simulink model "Fig7_Control_RLcurrent_PI"  (R2022a)
settings: Solver=FixedStepAuto  StartTime=0.0  StopTime=0.4  FixedStep=1e-4  RelTol=1e-3
InitFcn:
  | KpKiDesign
StartFcn:
  | KpKiDesign
values from neighbouring files (symbols this model uses):
  Ki = R/tau    (= 5)    [Fig17_drawBodeCPminusP.m]    (also in Fig22_drawBodePIctrl.m = [0.1;  0;      0;      0.1; 0.1]; KpKiDesign.m)
  Kp = L/tau    (= 0.2)    [Fig17_drawBodeCPminusP.m]    (also in Fig22_drawBodePIctrl.m = [0;    0.01;   0.1;    0.1; 0.01]; KpKiDesign.m)
  L = 4e-3    (= 0.004)    [Fig17_drawBodeCPminusP.m]    (also in KpKiDesign.m; RLCurcuitParam.m)
  R = 0.1    [Fig17_drawBodeCPminusP.m]    (also in KpKiDesign.m; RLCurcuitParam.m)
settings Model: Creator=r720r  LastModifiedBy=r720r

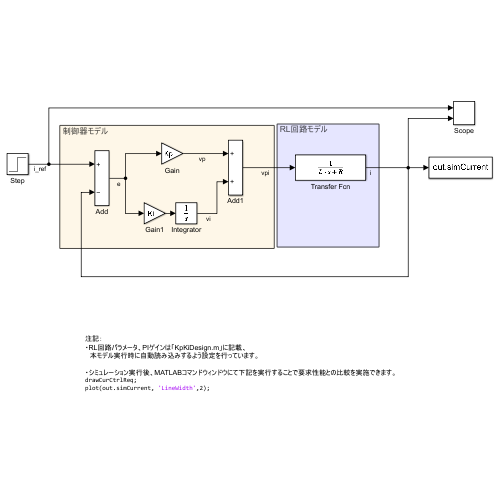
[thumbnail: Simulink's stored preview of the top-level diagram]
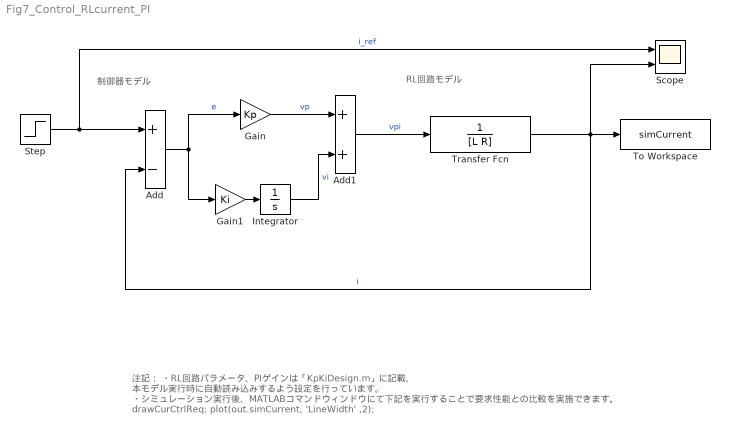
== system Fig7_Control_RLcurrent_PI ==
  note: RL回路モデル
  note: 制御器モデル
  note: 注記：
      | ・RL回路パラメータ、PIゲインは「KpKiDesign.m」に記載、
      | 本モデル実行時に自動読み込みするよう設定を行っています。
      |
      | ・シミュレーション実行後、MATLABコマンドウィンドウにて下記を実行することで要求性能との比較を実施できます。
      | drawCurCtrlReq;
      | plot(out.simCurrent, 'LineWidth' ,2);
  Add : Sum  Inputs=+-
  Add1 : Sum
  Gain : Gain  Gain=Kp
  Gain1 : Gain  Gain=Ki
  Integrator : Integrator
  Scope : Scope  NumInputPorts=2
  Step : Step  Time=0  SampleTime=0
  To Workspace : ToWorkspace  VariableName=simCurrent  SaveFormat=Timeseries  SampleTime=-1
  Transfer Fcn : TransferFcn  Denominator=[L R]
  wires:
  Step/1 -> Scope/1, Add/1  "i_ref"
  Add/1 -> Gain/1, Gain1/1  "e"
  Transfer Fcn/1 -> To Workspace/1, Add/2, Scope/2  "i"
  Gain1/1 -> Integrator/1
  Integrator/1 -> Add1/2  "vi"
  Gain/1 -> Add1/1  "vp"
  Add1/1 -> Transfer Fcn/1  "vpi"
